simulink subsystem "Plot_Data"  (R2025a)
settings: Solver=VariableStepAuto  StartTime=0.0  StopTime=10.0  RelTol=1e-3
undefined symbols (not defined in the file): gcs
settings Model: Creator=gurt1  LastModifiedBy=17036

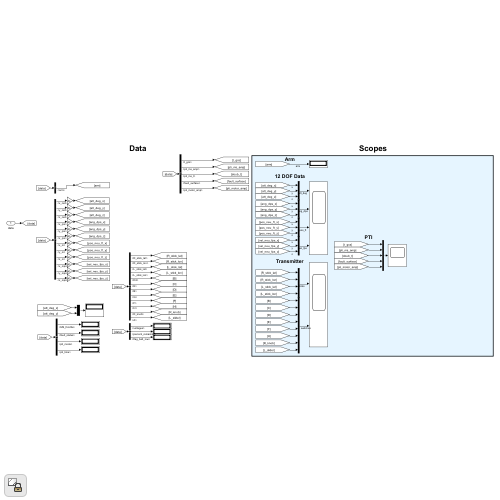
[thumbnail: Simulink's stored preview of the top-level diagram]
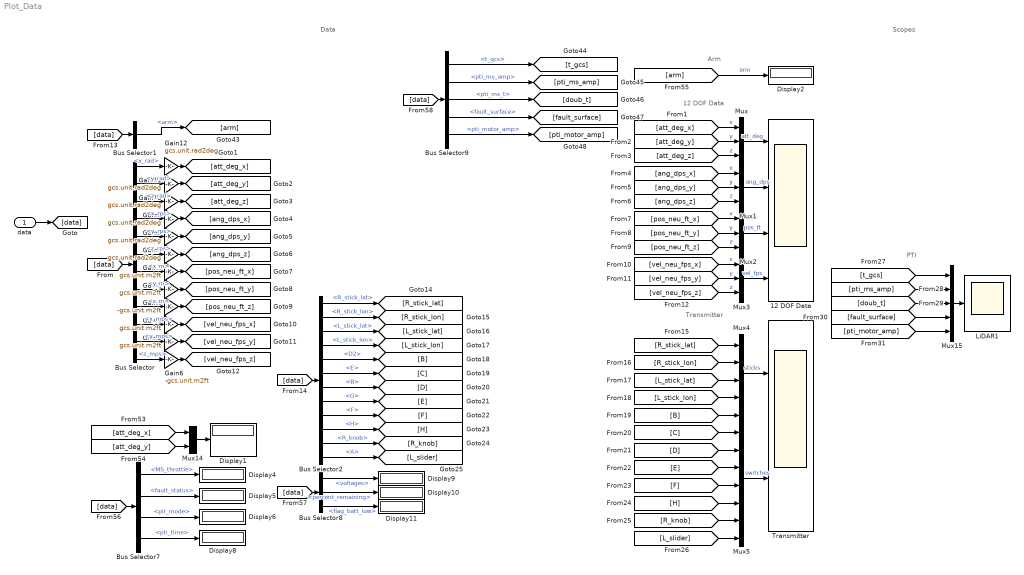
== system Plot_Data ==
  note: Scopes
  note: 12 DOF Data
  note: Transmitter
  note: Arm
  note: Data
  note: PTI
  data : Inport
  12 DOF Data : Scope  NumInputPorts=4
      settings: TimeSpan=100  ActiveDisplayYMinimum=-1  ActiveDisplayYMaximum=1
  Bus Selector : BusSelector  OutputSignals=VehicleAttitude.x_rad,VehicleAttitude.y_rad,VehicleAttitude.z_rad,VehicleAngularVelocity.x_rps,VehicleAngularVelocity.y_rps,VehicleAngularVelocity.z_rps,VehicleLocalPosition.x_m,VehicleLocalPosition.y_m,VehicleLocalPosition.z_m,VehicleLocalPosition.x_mps,VehicleLocalPosition.y_mps,VehicleLocalPosition.z_mps
  Bus Selector1 : BusSelector  OutputSignals=DebugArray.arm.arm
  Bus Selector2 : BusSelector  OutputSignals=DebugArray.rc_cmds.R_stick_lat,DebugArray.rc_cmds.R_stick_lon,DebugArray.rc_cmds.L_stick_lat,DebugArray.rc_cmds.L_stick_lon,DebugArray.rc_cmds.D2,DebugArray.rc_cmds.E,DebugArray.rc_cmds.B,DebugArray.rc_cmds.G,DebugArray.rc_cmds.F,DebugArray.rc_cmds.H,DebugArray.rc_cmds.R_knob,DebugArray.rc_cmds.A
  Bus Selector7 : BusSelector  OutputSignals=DebugArray.modes.MS_throttle,DebugArray.modes.fault_status,DebugArray.modes.pit_mode,DebugArray.modes.pti_time
  Bus Selector8 : BusSelector  OutputSignals=BatteryStatus.voltages,BatteryStatus.percent_remaining,BatteryStatus.flag_batt_low
  Bus Selector9 : BusSelector  OutputSignals=DebugArray.ol_pti.t_gcs,DebugArray.ol_pti.pti_ms_amp,DebugArray.ol_pti.pti_ms_t,DebugArray.ol_pti.fault_surface,DebugArray.ol_pti.pti_motor_amp
  Display{1..2,4..6,8..11} (9 alike) : Display
  Gain{1..2,4..5} (4 alike) : Gain  Gain=gcs.unit.m2ft
  Gain{7..12} (6 alike) : Gain  Gain=gcs.unit.rad2deg
  Gain3 : Gain  Gain=-gcs.unit.m2ft
  Gain6 : Gain  Gain=-gcs.unit.m2ft
  LiDAR1 : Scope
      settings: TimeSpan=100  Title=PX4 vs LiDAR Altitude  ActiveDisplayYMinimum=-1.25  ActiveDisplayYMaximum=11.25  DataLoggingVariableName=ScopeData6
  Mux{,1..3} (4 alike) : Mux  Inputs=3
  Mux14 : Mux  Inputs=2
  Mux15 : Mux  Inputs=5
  Mux4 : Mux
  Mux5 : Mux  Inputs=8
  Transmitter : Scope  NumInputPorts=2
      settings: TimeSpan=100  ActiveDisplayYMinimum=-1  ActiveDisplayYMaximum=1
  wires:
  [data] -> Bus Selector/1
  Bus Selector/1 -> Gain12/1  "<x_rad>"
  Bus Selector/2 -> Gain11/1  "<y_rad>"
  Bus Selector/3 -> Gain10/1  "<z_rad>"
  Bus Selector/4 -> Gain9/1  "<x_rps>"
  Bus Selector/5 -> Gain8/1  "<y_rps>"
  Bus Selector/6 -> Gain7/1  "<z_rps>"
  Bus Selector/7 -> Gain1/1  "<x_m>"
  Bus Selector/8 -> Gain2/1  "<y_m>"
  Bus Selector/9 -> Gain3/1  "<z_m>"
  Bus Selector/10 -> Gain4/1  "<x_mps>"
  Bus Selector/11 -> Gain5/1  "<y_mps>"
  Bus Selector/12 -> Gain6/1  "<z_mps>"
  Mux/1 -> 12 DOF Data/1  "att_deg"
  Mux1/1 -> 12 DOF Data/2  "ang_dps"
  Mux3/1 -> 12 DOF Data/4  "vel_fps"
  Mux2/1 -> 12 DOF Data/3  "pos_ft"
  [att_deg_x] -> Mux/1  "x"
  [att_deg_y] -> Mux/2  "y"
  [att_deg_z] -> Mux/3  "z"
  [ang_dps_x] -> Mux1/1  "x"
  [ang_dps_y] -> Mux1/2  "y"
  [ang_dps_z] -> Mux1/3  "z"
  [pos_neu_ft_x] -> Mux2/1  "x"
  [pos_neu_ft_y] -> Mux2/2  "y"
  [pos_neu_ft_z] -> Mux2/3  "z"
  [vel_neu_fps_x] -> Mux3/1  "x"
  [vel_neu_fps_y] -> Mux3/2  "y"
  [vel_neu_fps_z] -> Mux3/3  "z"
  [data] -> Bus Selector1/1
  [data] -> Bus Selector2/1
  Bus Selector2/1 -> [R_stick_lat]  "<R_stick_lat>"
  Bus Selector2/2 -> [R_stick_lon]  "<R_stick_lon>"
  Bus Selector2/3 -> [L_stick_lat]  "<L_stick_lat>"
  Bus Selector2/4 -> [L_stick_lon]  "<L_stick_lon>"
  Bus Selector2/5 -> [B]  "<D2>"
  Bus Selector2/6 -> [C]  "<E>"
  Bus Selector2/7 -> [D]  "<B>"
  Bus Selector2/8 -> [E]  "<G>"
  Bus Selector2/9 -> [F]  "<F>"
  Bus Selector2/10 -> [H]  "<H>"
  Bus Selector2/11 -> [R_knob]  "<R_knob>"
  Bus Selector2/12 -> [L_slider]  "<A>"
  Mux4/1 -> Transmitter/1  "sticks"
  Mux5/1 -> Transmitter/2  "switches"
  [R_stick_lat] -> Mux4/1
  [R_stick_lon] -> Mux4/2
  [L_stick_lat] -> Mux4/3
  [L_stick_lon] -> Mux4/4
  [B] -> Mux5/1
  [C] -> Mux5/2
  [D] -> Mux5/3
  [E] -> Mux5/4
  [F] -> Mux5/5
  [H] -> Mux5/6
  [R_knob] -> Mux5/7
  [L_slider] -> Mux5/8
  Gain1/1 -> [pos_neu_ft_x]
  Gain2/1 -> [pos_neu_ft_y]
  Gain3/1 -> [pos_neu_ft_z]
  Gain4/1 -> [vel_neu_fps_x]
  Gain5/1 -> [vel_neu_fps_y]
  Gain6/1 -> [vel_neu_fps_z]
  Gain7/1 -> [ang_dps_z]
  Gain8/1 -> [ang_dps_y]
  Gain9/1 -> [ang_dps_x]
  Gain10/1 -> [att_deg_z]
  Gain11/1 -> [att_deg_y]
  Gain12/1 -> [att_deg_x]
  [att_deg_x] -> Mux14/1
  [att_deg_y] -> Mux14/2
  Mux14/1 -> Display1/1
  Bus Selector1/1 -> [arm]  "<arm>"
  [arm] -> Display2/1  "arm"
  [data] -> Bus Selector7/1
  Bus Selector7/1 -> Display4/1  "<MS_throttle>"
  Bus Selector7/2 -> Display5/1  "<fault_status>"
  Bus Selector7/3 -> Display6/1  "<pit_mode>"
  Bus Selector7/4 -> Display8/1  "<pti_time>"
  [data] -> Bus Selector8/1
  Bus Selector8/1 -> Display9/1  "<voltages>"
  Bus Selector8/2 -> Display10/1  "<percent_remaining>"
  [data] -> Bus Selector9/1
  Bus Selector9/1 -> [t_gcs]  "<t_gcs>"
  Bus Selector9/2 -> [pti_ms_amp]  "<pti_ms_amp>"
  Bus Selector9/3 -> [doub_t]  "<pti_ms_t>"
  Bus Selector9/4 -> [fault_surface]  "<fault_surface>"
  Bus Selector9/5 -> [pti_motor_amp]  "<pti_motor_amp>"
  Mux15/1 -> LiDAR1/1
  [t_gcs] -> Mux15/1
  [pti_motor_amp] -> Mux15/5
  [fault_surface] -> Mux15/4
  [doub_t] -> Mux15/3
  [pti_ms_amp] -> Mux15/2
  Bus Selector8/3 -> Display11/1  "<flag_batt_low>"
  data/1 -> [data]
